simulink model "sldemo_discretedrivingcycle"  (R2021a)
settings: Solver=FixedStepDiscrete  StartTime=0.0  StopTime=1e5  MaxStep=1  RelTol=1e-3  EnableMultiTasking=on
undefined symbols (not defined in the file): DiscIntNeverNeededParam
libraries: drivingcycle_lib x1
settings Model: Creator=e102261  LastModifiedBy=secch
settings SolverCC: AlgebraicLoopSolver=TrustRegion
settings DataIOCC: LimitDataPoints=on  SaveFormat=Array  SaveOutput=off  SignalLogging=off  DSMLogging=off  SaveTime=off  ReturnWorkspaceOutputs=off
settings OptimizationCC: ExpressionDepthLimit=2147483647  LifeSpan=inf
settings DebuggingCC: UnderspecifiedInitializationDetection=Classic  MergeDetectMultiDrivingBlocksExec=none  SolverPrmCheckMsg=warning  MultiTaskDSMMsg=warning  MultiTaskCondExecSysMsg=none  FcnCallInpInsideContextMsg=warning  StateNameClashWarn=warning  SFUnexpectedBacktrackingDiag=warning  SFNoUnconditionalDefaultTransitionDiag=warning  SFExecutionAtInitializationDiag=none  SFMachineParentedDataDiag=warning  ArithmeticOperatorsInVariantConditions=warning
settings HardwareCC: ProdBitPerPointer=32  ProdBitPerSizeT=32  ProdBitPerPtrDiffT=32  ProdLargestAtomicFloat=None  ProdIntDivRoundTo=Undefined  ProdEndianess=Unspecified  ProdWordSize=32  ProdHWDeviceType=32-bit Generic
settings ModelReferenceCC: PropagateSignalLabelsOutOfModel=off
settings SFSimCC: SimUseLocalCustomCode=off  CustomCodeUndefinedFunction=UseInterfaceOnly
settings RTWCC: RTWUseLocalCustomCode=off
settings CodeAppCC: StateflowObjectComments=on
settings GRTTargetCC: TargetLangStandard=C89/C90 (ANSI)
settings ConfigComp: CovMetricSettings=dw  CovSaveCumulativeToWorkspaceVar=on  CovSaveSingleToWorkspaceVar=on  CovExternalEMLEnable=off

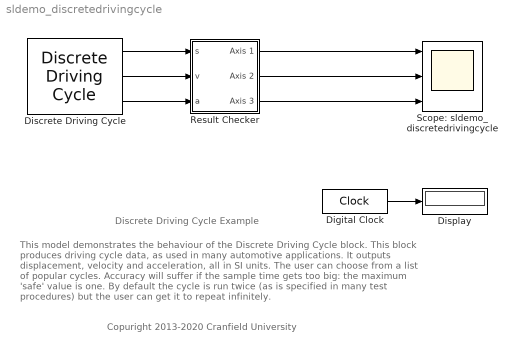
== system sldemo_discretedrivingcycle ==
  note: Discrete Driving Cycle Example
  note: This model demonstrates the behaviour of the Discrete Driving Cycle block.
      | This block produces driving cycle data, as used in many automotive applications.
      | It outputs displacement, velocity and acceleration, all in SI units.  The user can
      | choose from a list of popular cycles.  Accuracy will suffer if the sample time gets
      | too big: the maximum 'safe' value is one.  By default the cycle is run twice (as
      | is specified in many test procedures) but the user can get it to repeat infinitely.
  note: Copuright 2013-2020 Cranfield University
  Digital Clock : DigitalClock
  Discrete Driving Cycle : drivingcycle_lib/Discrete Driving Cycle  CycleName=WLTP class 3  CycleRepeatsForever=off  SampleTime=1
      settings: SourceProductName=Driving Cycle Blockset
  Display : Display
  Result Checker : Subsystem
  Scope: sldemo_discretedrivingcycle : Scope  NumInputPorts=3
      settings: AttributesFormatString=|
      | please use scope's axis autoscaling
      | button after simulation
  wires:
  Result Checker/1(Axis 1) -> Scope: sldemo_discretedrivingcycle/1
  Result Checker/2(Axis 2) -> Scope: sldemo_discretedrivingcycle/2
  Result Checker/3(Axis 3) -> Scope: sldemo_discretedrivingcycle/3
  Discrete Driving Cycle/1 -> Result Checker/1(s)
  Discrete Driving Cycle/3 -> Result Checker/3(a)
  Digital Clock/1 -> Display/1
  Discrete Driving Cycle/2 -> Result Checker/2(v)

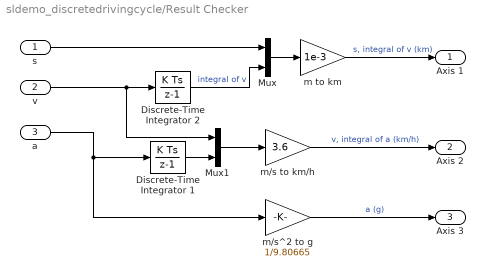
== system sldemo_discretedrivingcycle/Result Checker ==
  s : Inport
  v : Inport  Port=2
  a : Inport  Port=3
  Discrete-Time Integrator 1 : DiscreteIntegrator  SampleTime=-1  ICPrevOutput=DiscIntNeverNeededParam  ICPrevScaledInput=DiscIntNeverNeededParam
  Discrete-Time Integrator 2 : DiscreteIntegrator  SampleTime=-1  ICPrevOutput=DiscIntNeverNeededParam  ICPrevScaledInput=DiscIntNeverNeededParam
  Mux : Mux  Inputs=2
  Mux1 : Mux  Inputs=2
  m to km : Gain  Gain=1e-3
  m/s to km/h : Gain  Gain=3.6
  m/s^2 to g : Gain  Gain=1/9.80665
  Axis 1 : Outport
  Axis 2 : Outport  Port=2
  Axis 3 : Outport  Port=3
  wires:
  m/s^2 to g/1 -> Axis 3/1  "a (g)"
  m/s to km/h/1 -> Axis 2/1  "v, integral of a (km/h)"
  m to km/1 -> Axis 1/1  "s, integral of v (km)"
  s/1 -> Mux/1
  a/1 -> Discrete-Time Integrator 1/1, m/s^2 to g/1
  v/1 -> Discrete-Time Integrator 2/1, Mux1/1
  Mux1/1 -> m/s to km/h/1
  Discrete-Time Integrator 2/1 -> Mux/2  "integral of v"
  Discrete-Time Integrator 1/1 -> Mux1/2
  Mux/1 -> m to km/1
